simulink model "beapil"  (Simulink 3.00)
settings: Solver=ode45  StartTime=0  StopTime=15  RelTol=1e-3
values from neighbouring files (symbols this model uses):
  alg = [-1.28411898435  0.976398373806; -6.85493241844  -3.02919350607]    [beadata.mat]
  blg = [-0.0929373395416 -10.6009202936]    [beadata.mat]
libraries: simulink3 x4, pil x4
settings Model: SaveTime=off  TimeSaveName=t  SaveOutput=off  LastModifiedBy=campa

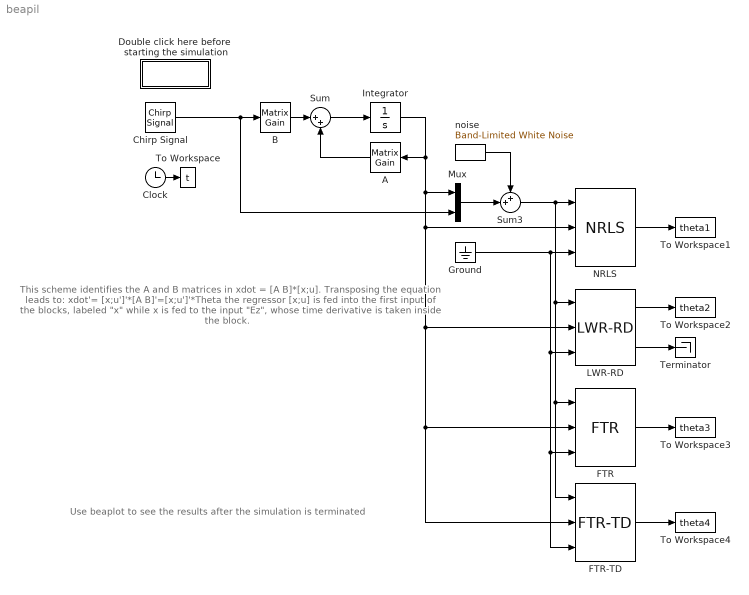
== system beapil ==
  note: Use beaplot to see the results
      | after the simulation is terminated
  note: This scheme identifies the A and B
      | matrices in xdot = [A B]*[x;u].
      |
      | Transposing the equation leads to:
      | xdot'= [x;u']'*[A B]'=[x;u']'*Theta
      | the regressor [x;u] is fed into the
      | first input of the blocks, labeled "x"
      | while x is fed to the input "Ez",
      | whose time derivative is taken
      | inside the block.
  A : simulink3/Math/Matrix Gain  Orientation=left  K=alg
  B : simulink3/Math/Matrix Gain  K=blg
  Chirp Signal : simulink3/Sources/Chirp Signal  f1=0.1  T=100  f2=1
  Clock : Clock
      settings: DisplayTime=off  Decimation=10
  Double click here before  starting the simulation : Subsystem
      settings: OpenFcn=load beadata;
      mask Display: disp('Load Model')
  FTR : pil/Only Theta/FTR  ths=[3 2]  w=2*pi*linspace(0.02,1.8,32)'  T=0.02
  FTR-TD : pil/Only Theta/FTR-TD  ths=[3 2]  w=2*pi*linspace(0.02,1.8,32)'  T=0.02
  Ground : Ground
  Integrator : Integrator  ExternalReset=none  InitialConditionSource=internal  InitialCondition=0  LimitOutput=off  UpperSaturationLimit=inf  LowerSaturationLimit=-inf  ShowSaturationPort=off  ShowStatePort=off  AbsoluteTolerance=auto
  LWR-RD : pil/Theta & Cov/LWR-RD  ths=[3 2]  n=50  sig=1  Tol=1e-6  x0=1  T=0.02
  Mux : Mux  Inputs=2
  NRLS : pil/Only Theta/NRLS  ths=[3 2]  lam=0.99  T=0.02
  Sum : Sum  Inputs=|++  SaturateOnIntegerOverflow=on
  Sum3 : Sum  Inputs=++|  SaturateOnIntegerOverflow=on
  Terminator : Terminator
  To Workspace : ToWorkspace  VariableName=t  SampleTime=0.02  SaveFormat=Matrix
  To Workspace1 : ToWorkspace  VariableName=theta1  SampleTime=0.02  SaveFormat=Matrix
  To Workspace2 : ToWorkspace  VariableName=theta2  SampleTime=0.02  SaveFormat=Matrix
  To Workspace3 : ToWorkspace  VariableName=theta3  SampleTime=0.02  SaveFormat=Matrix
  To Workspace4 : ToWorkspace  VariableName=theta4  SampleTime=0.02  SaveFormat=Matrix
  noise : simulink3/Sources/Band-Limited White Noise  Cov=[1 1 1]*1e-5  Ts=0.02  seed=[1 2 3]
  wires:
  B/1 -> Sum/1
  Clock/1 -> To Workspace/1
  NRLS/1 -> To Workspace1/1
  FTR/1 -> To Workspace3/1
  Ground/1 -> NRLS/3, LWR-RD/3, FTR/3, FTR-TD/3
  Sum3/1 -> NRLS/1, LWR-RD/1, FTR/1, FTR-TD/1
  FTR-TD/1 -> To Workspace4/1
  LWR-RD/2 -> Terminator/1
  LWR-RD/1 -> To Workspace2/1
  noise/1 -> Sum3/1
  Mux/1 -> Sum3/2
  Integrator/1 -> A/1, Mux/1, NRLS/2, LWR-RD/2, FTR/2, FTR-TD/2
  Sum/1 -> Integrator/1
  Chirp Signal/1 -> B/1, Mux/2
  A/1 -> Sum/2

== system beapil/Double click here before  starting the simulation ==
